simulink model "PI_Retour_Etat_LQG"  (R2024a)
settings: Solver=VariableStepAuto  StartTime=0.0  StopTime=50  RelTol=1e-3
undefined symbols (not defined in the file): A, A_kal, B, B_kal, C_kal, D_kal, K_lqr, Ts, x0
settings Model: Creator=DELL  LastModifiedBy=DELL

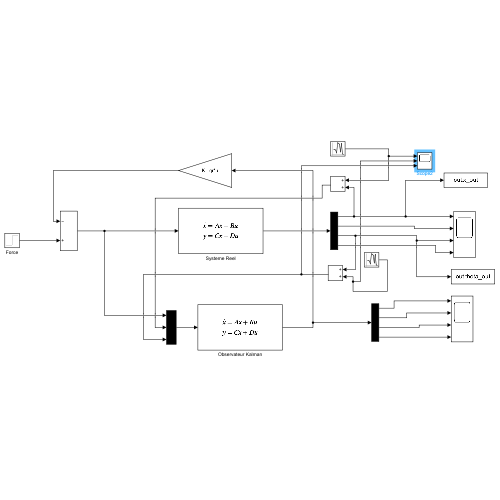
[thumbnail: Simulink's stored preview of the top-level diagram]
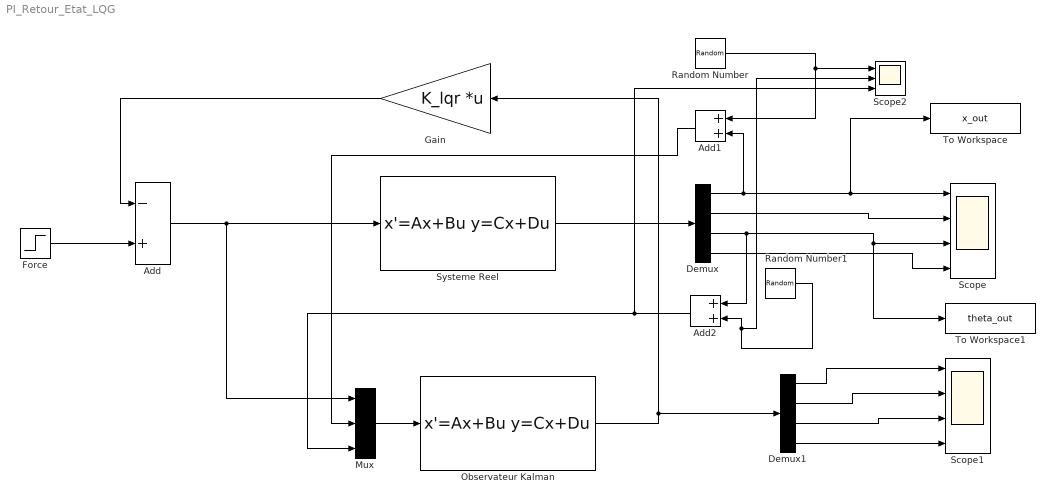
== system PI_Retour_Etat_LQG ==
  Add : Sum  Inputs=-+
  Add1 : Sum
  Add2 : Sum
  Demux : Demux
  Demux1 : Demux
  Force : Step  Time=5  After=15  SampleTime=Ts
  Gain : Gain  Gain=K_lqr  Multiplication=Matrix(K*u)
  Mux : Mux  Inputs=3
  Observateur Kalman : StateSpace  A=A_kal  B=B_kal  C=C_kal  D=D_kal  InitialCondition=[0 0 0 0]
  Random Number : RandomNumber  Variance=0.001  SampleTime=Ts
  Random Number1 : RandomNumber  Variance=0.001  SampleTime=Ts
  Scope : Scope  NumInputPorts=4
  Scope1 : Scope  NumInputPorts=4
  Scope2 : Scope  NumInputPorts=3
  Systeme Reel : StateSpace  A=A  B=B  C=eye(4);  D=zeros(4,1);  InitialCondition=x0
  To Workspace : ToWorkspace  VariableName=x_out  SaveFormat=Timeseries  SampleTime=-1
  To Workspace1 : ToWorkspace  VariableName=theta_out  SaveFormat=Timeseries  SampleTime=-1
  wires:
  Demux/1 -> Add1/2, To Workspace/1, Scope/1
  Gain/1 -> Add/1
  Systeme Reel/1 -> Demux/1
  Demux/2 -> Scope/2
  Demux/3 -> Add2/1, To Workspace1/1, Scope/3
  Add/1 -> Mux/1, Systeme Reel/1
  Observateur Kalman/1 -> Demux1/1, Gain/1
  Demux1/1 -> Scope1/1
  Mux/1 -> Observateur Kalman/1
  Demux1/2 -> Scope1/2
  Demux1/3 -> Scope1/3
  Demux1/4 -> Scope1/4
  Demux/4 -> Scope/4
  Force/1 -> Add/2
  Random Number/1 -> Add1/1, Scope2/1
  Random Number1/1 -> Scope2/2, Add2/2
  Add2/1 -> Scope2/3, Mux/3
  Add1/1 -> Mux/2
